simulink model "CEGR_TestBench_10kW_SimplifiedEGR_v01"  (R2025b)
settings: Solver=ode4  StartTime=0.0  StopTime=120  FixedStep=0.02  RelTol=1e-3
undefined symbols (not defined in the file): CaseBoundaryParam_simplified, CoolingCurveParam_simplified, dt_s_simplified, EGRInitialNode_simplified, PhysicalParam_simplified, StackInitialState_simplified, StackModelParam_simplified
settings Model: Creator=ADMIN  LastModifiedBy=ADMIN

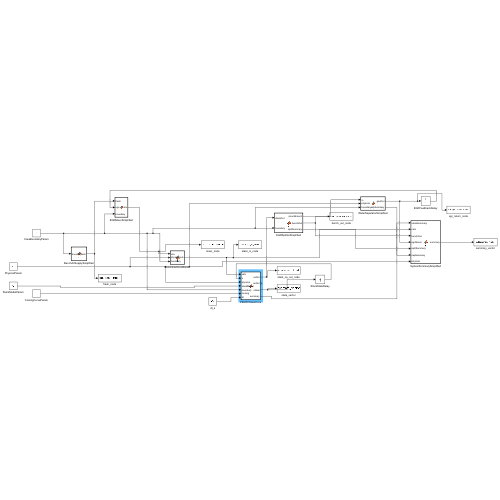
[thumbnail: Simulink's stored preview of the top-level diagram]
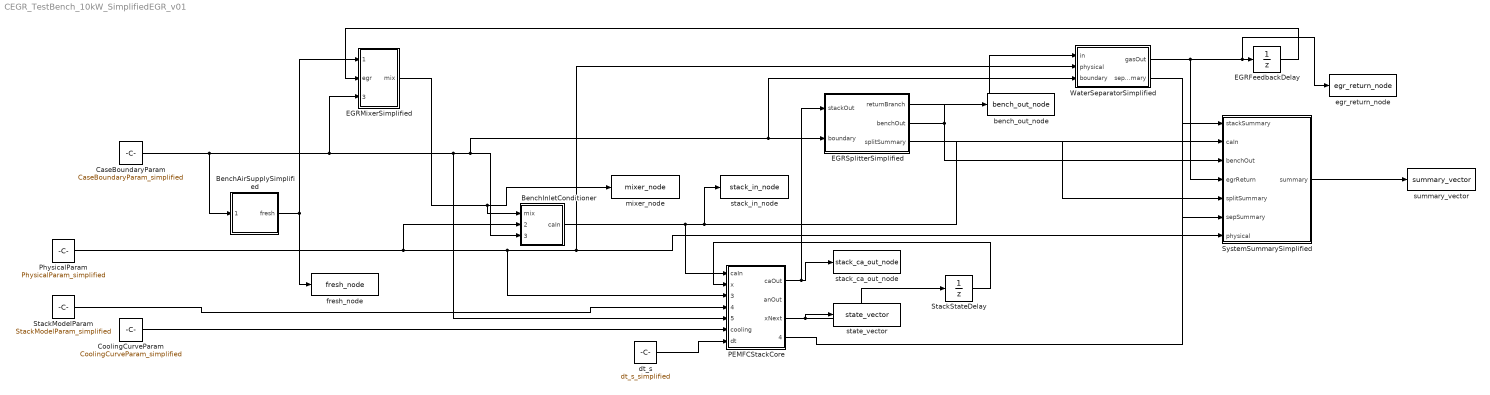
== system CEGR_TestBench_10kW_SimplifiedEGR_v01 ==
  BenchAirSupplySimplified : MATLAB Function  TreatAsAtomicUnit=on
  BenchInletConditioner : MATLAB Function  TreatAsAtomicUnit=on
  CaseBoundaryParam : Constant  Value=CaseBoundaryParam_simplified
  CoolingCurveParam : Constant  Value=CoolingCurveParam_simplified
  EGRFeedbackDelay : UnitDelay  InitialCondition=EGRInitialNode_simplified  SampleTime=dt_s_simplified
  EGRMixerSimplified : MATLAB Function  TreatAsAtomicUnit=on
  EGRSplitterSimplified : MATLAB Function  TreatAsAtomicUnit=on
  PEMFCStackCore : MATLAB Function  TreatAsAtomicUnit=on
  PhysicalParam : Constant  Value=PhysicalParam_simplified
  StackModelParam : Constant  Value=StackModelParam_simplified
  StackStateDelay : UnitDelay  InitialCondition=StackInitialState_simplified  SampleTime=dt_s_simplified
  SystemSummarySimplified : MATLAB Function  TreatAsAtomicUnit=on
  WaterSeparatorSimplified : MATLAB Function  TreatAsAtomicUnit=on
  bench_out_node : ToWorkspace  VariableName=bench_out_node  SaveFormat=Structure With Time
  dt_s : Constant  Value=dt_s_simplified
  egr_return_node : ToWorkspace  VariableName=egr_return_node  SaveFormat=Structure With Time
  fresh_node : ToWorkspace  VariableName=fresh_node  SaveFormat=Structure With Time
  mixer_node : ToWorkspace  VariableName=mixer_node  SaveFormat=Structure With Time
  stack_ca_out_node : ToWorkspace  VariableName=stack_ca_out_node  SaveFormat=Structure With Time
  stack_in_node : ToWorkspace  VariableName=stack_in_node  SaveFormat=Structure With Time
  state_vector : ToWorkspace  VariableName=state_vector  SaveFormat=Structure With Time
  summary_vector : ToWorkspace  VariableName=summary_vector  SaveFormat=Structure With Time
  wires:
  PhysicalParam/1 -> WaterSeparatorSimplified/2(physical), SystemSummarySimplified/7(physical), PEMFCStackCore/3(physical), BenchInletConditioner/2(physical)
  CaseBoundaryParam/1 -> PEMFCStackCore/5(boundary), EGRSplitterSimplified/2(boundary), WaterSeparatorSimplified/3(boundary), BenchInletConditioner/3(boundary), EGRMixerSimplified/3(boundary), BenchAirSupplySimplified/1(boundary)
  StackModelParam/1 -> PEMFCStackCore/4(stackModel)
  CoolingCurveParam/1 -> PEMFCStackCore/6(cooling)
  StackStateDelay/1 -> PEMFCStackCore/2(x)
  BenchAirSupplySimplified/1(fresh) -> EGRMixerSimplified/1(fresh), fresh_node/1
  EGRFeedbackDelay/1 -> EGRMixerSimplified/2(egr)
  EGRMixerSimplified/1(mix) -> mixer_node/1, BenchInletConditioner/1(mix)
  BenchInletConditioner/1(caIn) -> SystemSummarySimplified/2(caIn), stack_in_node/1, PEMFCStackCore/1(caIn)
  PEMFCStackCore/1(caOut) -> EGRSplitterSimplified/1(stackOut), stack_ca_out_node/1
  WaterSeparatorSimplified/1(gasOut) -> EGRFeedbackDelay/1, egr_return_node/1, SystemSummarySimplified/4(egrReturn)
  PEMFCStackCore/3(xNext) -> StackStateDelay/1, state_vector/1
  PEMFCStackCore/4(summary) -> SystemSummarySimplified/1(stackSummary)
  EGRSplitterSimplified/2(benchOut) -> bench_out_node/1, SystemSummarySimplified/3(benchOut)
  EGRSplitterSimplified/3(splitSummary) -> SystemSummarySimplified/5(splitSummary)
  WaterSeparatorSimplified/2(sepSummary) -> SystemSummarySimplified/6(sepSummary)
  SystemSummarySimplified/1(summary) -> summary_vector/1
  EGRSplitterSimplified/1(returnBranch) -> WaterSeparatorSimplified/1(in)
  dt_s/1 -> PEMFCStackCore/7(dt)

== matlab function CEGR_TestBench_10kW_SimplifiedEGR_v01/EGRMixerSimplified ==
  data: fresh input; mix output; egr input; boundary input
function mix = f(fresh, egr, boundary)
% EGRMixerSimplified
% 功能：把台架新鲜供气与延迟回流 EGR 混合，并生成目标入堆质量流量。
% 位置：BenchAirSupplySimplified 与 BenchInletConditioner 之间。
% 输入 fresh：新鲜供气 7x1 向量，fresh(1:4) 在此处按组分质量分数使用。
% 输入 egr：来自 EGRFeedbackDelay 的回流 7x1 向量，egr(1:4) 为可回流质量流量。
% 输入 boundary：CaseBoundaryParam_simplified，本模块使用 boundary(4) 入堆目标总质量流量。
% 输出 mix：7x1 混合气向量，mix(1:4) 为质量流量，供 BenchInletConditioner 使用。
%#codegen

mTarget = boundary(4);
assert(mTarget > 0);
assert(all(fresh(1:4) >= 0));
assert(all(egr(1:4) >= 0));
assert(fresh(5) >= -40 && fresh(5) <= 120 && fresh(6) > 0);

% 新鲜气输入来自 BenchAirSupplySimplified，前四项应能归一化为组分比例。
freshMassBasis = sum(fresh(1:4));
assert(freshMassBasis > 0);
freshFrac = fresh(1:4) / freshMassBasis;

% EGR 可用量取回流气相质量流量。液态水只作为组分携带，不用于决定回流气体替代量。
availableEgrGas = sum(egr(1:3));
egrTotalBasis = sum(egr(1:4));

% 最多让 EGR 替代 95% 的目标入堆流量，保留至少 5% 新鲜气补充。
% 这是当前简化模型的物理/数值边界，不是输入数据纠错。
egrToMix = min(availableEgrGas, 0.95 * mTarget);
freshMakeup = mTarget - egrToMix;

if egrToMix > 0
    assert(egrTotalBasis > 0);
    assert(egr(5) >= -40 && egr(5) <= 120 && egr(6) > 0);
    egrFrac = egr(1:4) / egrTotalBasis;
else
    egrFrac = zeros(4, 1);
end

mix = zeros(7, 1);
mix(1:4) = freshMakeup * freshFrac + egrToMix * egrFrac;
mixedMass = freshMakeup + egrToMix;
assert(mixedMass > 0);
mix(5) = (fresh(5) * freshMakeup + egr(5) * egrToMix) / mixedMass;
mix(6) = fresh(6);
mix(7) = double(mix(4) > 1e-12);
end

== matlab function CEGR_TestBench_10kW_SimplifiedEGR_v01/BenchAirSupplySimplified ==
  data: fresh output; boundary input
function fresh = f(boundary)
% BenchAirSupplySimplified
% 功能：把台架新鲜空气边界转换为模型统一气体向量 fresh。
% 位置：气路最外侧的新鲜供气端，输出进入 EGRMixerSimplified。
% 输入 boundary：CaseBoundaryParam_simplified 单工况边界向量。
%   boundary(2) = stack_in_p_abs_kPa，阴极入口绝压边界。
%   boundary(3) = stack_in_T_C，阴极入口温度边界。
%   boundary(5:7) = cathode_supply_wO2/wN2/wH2O，由台架供气 p/T/RH 换算得到的湿空气质量分数。
% 输出 fresh：7x1 气体向量，约定为 [O2; N2; H2O_vapor; H2O_liquid; T_C; p_kPa; wetFlag]。
% 注意：fresh(1:3) 在这里是归一化质量分数，不是质量流量；实际入堆总流量由后续混合器使用 boundary(4) 施加。
%#codegen

% 供气质量分数是输入边界，不能在模型里静默截断；负值应暴露为数据或映射错误。
wO2 = boundary(5);
wN2 = boundary(6);
wV = boundary(7);
assert(wO2 >= 0 && wN2 >= 0 && wV >= 0);

% 允许微小数值误差下的归一化，但质量分数和必须为正。
massFractionSum = wO2 + wN2 + wV;
assert(massFractionSum > 0);

% 新鲜供气支路不携带液态水，wetFlag=0 表示未发生冷凝/液水携带。
fresh = [
    wO2 / massFractionSum
    wN2 / massFractionSum
    wV / massFractionSum
    0
    boundary(3)
    boundary(2)
    0
    ];
end

== matlab function CEGR_TestBench_10kW_SimplifiedEGR_v01/BenchInletConditioner ==
  data: mix input; caIn output; physical input; boundary input
function caIn = f(mix, physical, boundary)
% BenchInletConditioner
% 功能：把混合器输出整理为电堆阴极入口气体向量 caIn。
% 位置：EGRMixerSimplified 与 PEMFCStackCore 之间，代表台架测得的入堆边界。
% 输入 mix：7x1 混合气向量，[O2; N2; H2O_vapor; H2O_liquid; T_C; p_kPa; wetFlag]。
% 输入 physical：通用物性向量，本模块使用 O2/N2/H2O 摩尔质量 physical(3:5)。
% 输入 boundary：CaseBoundaryParam_simplified，本模块使用 boundary(2) 入口绝压和 boundary(3) 入口温度。
% 输出 caIn：7x1 阴极入口向量，质量流量来自 mix，温度/压力强制采用实测入堆边界。
%#codegen

M_O2 = physical(3);
M_N2 = physical(4);
M_H2O = physical(5);
p = boundary(2);
T = boundary(3);

% 这些是硬输入/物性检查。异常值应暴露为参数或上游模块错误，不能静默修正。
assert(M_O2 > 0 && M_N2 > 0 && M_H2O > 0);
assert(p > 0);
assert(T >= -40 && T <= 120);
assert(all(mix(1:4) >= 0));

% 入口流量和组分沿用混合器输出；入口温压采用实验入堆边界。
caIn = mix;
caIn(5) = T;
caIn(6) = p;

% 依据入口温压计算可携带的饱和水蒸气质量流量。
% min(...,0.98*p) 是物理上限：水蒸气分压不能接近或超过总压。
pSat = min(sat_kPa(T), 0.98 * p);
nDry = caIn(1) / M_O2 + caIn(2) / M_N2;
assert(nDry > 0);
mVaporSat = pSat * nDry / (p - pSat) * M_H2O;

% 如果混合气在入口温压下超饱和，超出的水蒸气转为液态水。
if caIn(3) > mVaporSat
    caIn(4) = caIn(4) + caIn(3) - mVaporSat;
    caIn(3) = mVaporSat;
end
caIn(7) = double(caIn(4) > 1e-12);
end

function p = sat_kPa(T)
% Buck 饱和水蒸气压公式，T 单位 degC；调用前已检查适用温度范围。
p = 0.61121 * exp((18.678 - T / 234.5) * (T / (257.14 + T)));
end

== matlab function CEGR_TestBench_10kW_SimplifiedEGR_v01/PEMFCStackCore ==
  data: caIn input; caOut output; x input; physical input; stackModel input; anOut output; xNext output; summary output; boundary input; cooling input; dt input
function [caOut, anOut, xNext, summary] = f(caIn, x, physical, stackModel, boundary, cooling, dt)
% PEMFCStackCore
% 功能：电堆核心低维动态模型，计算阴极/阳极气体库存、膜水迁移、热平衡和单片电压。
% 输入 caIn：BenchInletConditioner 输出的阴极入口 7x1 向量，caIn(1:4) 为质量流量。
% 输入 x：StackStateDelay 反馈的状态向量 [mO2;mN2;mH2O_ca;mH2;mH2O_an;T_stack_C;mMem]。
% 输入 physical：物理常数向量 [R;F;M_O2;M_N2;M_H2O;M_H2;p_amb;T_amb]。
% 输入 stackModel：电堆结构、出口导纳、热参数、电压参数和膜水松弛参数。
% 输入 boundary：单工况边界；本模块使用电流、出口背压、阳极入口和冷却边界。
% 输入 cooling：冷却流量-换热系数曲线；dt：离散仿真步长。
% 输出 caOut/anOut：电堆阴极/阳极出口气体向量；输出 xNext：下一步状态；summary：诊断量。
%#codegen

% 参数解包。
R = physical(1); F = physical(2); M_O2 = physical(3); M_N2 = physical(4); M_H2O = physical(5); M_H2 = physical(6); pamb = physical(7); Tamb = physical(8);
N = stackModel(1); A = stackModel(2); Vca = stackModel(3); Van = stackModel(4); Kca = stackModel(5); Kan = stackModel(6); Cfc = stackModel(7); hCool = stackModel(8); hAmb = stackModel(9);
Eref = stackModel(10); Etemp = stackModel(11); theta1 = stackModel(12); theta2 = stackModel(13); theta3 = stackModel(14); theta4 = stackModel(15); sigmaPemCorrection = stackModel(16); Vtn = stackModel(17); tauMem = stackModel(18);
% 书籍活化极化经验式使用 theta1~theta4；欧姆项使用膜电导率公式。
% I_leak 固定为 0.01 A/cm2，只用于 log(j + I_leak) 避免零电流奇异。
jLeak = 0.01;
deltaCm = 0.0025; rhoMem = 1980.0; EW = 1.10;
I = boundary(1); pcBack = boundary(8); anFlow = boundary(12); anWH2 = boundary(13); anWV = boundary(14); panBack = boundary(15); Tcool = boundary(16); coolantFlow = boundary(17);

% 输入硬校验：这些是参数或边界错误，不能在核心模型里静默夹取。
assert(R > 0 && F > 0 && M_O2 > 0 && M_N2 > 0 && M_H2O > 0 && M_H2 > 0);
assert(pamb > 0 && Tamb >= -40 && Tamb <= 120);
assert(N > 0 && A > 0 && Vca > 0 && Van > 0 && Cfc > 0 && tauMem > 0);
assert(Kca >= 0 && Kan >= 0 && hCool >= 0 && hAmb >= 0);
assert(theta3 < 0 && theta4 >= 0 && jLeak >= 0);
assert(deltaCm > 0 && sigmaPemCorrection > 0 && rhoMem > 0 && EW > 0);
assert(I >= 0 && pcBack > 0 && panBack > 0 && anFlow > 0 && Tcool >= -40 && Tcool <= 120 && coolantFlow >= 0 && dt > 0);
assert(anWH2 >= 0 && anWH2 <= 1 && anWV >= 0 && anWV <= 1 && anWH2 + anWV <= 1.000001);
assert(numel(x) >= 6 && all(x(1:5) >= 0) && x(6) >= -40 && x(6) <= 120);
assert(all(caIn(1:4) >= 0) && caIn(5) >= -40 && caIn(5) <= 120 && caIn(6) > 0);
assert(sum(caIn(1:3)) > 0);

% 冷却换热系数：只有曲线启用且有效断点不少于 2 个时，才用流量插值覆盖默认 hCool。
hCoolEff = hCool;
nCool = floor((numel(cooling) - 1) / 2);
if nCool >= 2 && cooling(1) > 0.5
    hCoolEff = interp_hcool_flow(coolantFlow, cooling(2:1+nCool), cooling(2+nCool:1+2*nCool), hCool);
end

% 状态读取：正气体库存使用小正数下限只为避免除零；负状态已由上方断言拦截。
mO2 = max(x(1), 1e-12); mN2 = max(x(2), 1e-12); mV = x(3); mH2 = max(x(4), 1e-12); mVAn = x(5); T = x(6); TK = T + 273.15;
mMemPrev = 0;
if numel(x) >= 7
    mMemPrev = x(7);
end

% 阴极入口与反应源项。
mInCmd = sum(caIn(1:3)); mIn = mInCmd; wIn = caIn(1:3) / mInCmd;
mO2In = mIn * wIn(1); mN2In = mIn * wIn(2); mVIn = mIn * wIn(3);
mO2React = I * N / (4 * F) * M_O2; mH2React = I * N / (2 * F) * M_H2; mWater = I * N / (2 * F) * M_H2O;
lambdaO2 = (mO2In / M_O2) / max(I * N / (4 * F), 1e-12);
mH2In = anFlow * anWH2; mVAnIn = anFlow * anWV;
nInTot = mO2In / M_O2 + mN2In / M_N2 + mVIn / M_H2O;
pVInCa = caIn(6) * (mVIn / M_H2O) / max(nInTot, 1e-12);

% Pre 基准库存：先施加入堆流量、反应消耗和产水，但暂不施加跨膜水通量。
mO2Base = max(mO2 + dt * (mO2In - mO2React), 1e-12);
mN2Base = max(mN2 + dt * mN2In, 1e-12);
mVBaseAct = max(mV + dt * mVIn, 0);
mVBaseGas = max(mV + dt * (mVIn + mWater), 0);
mH2Base = max(mH2 + dt * (mH2In - mH2React), 1e-12);
mVAnBase = max(mVAn + dt * mVAnIn, 0);

% 膜含水量和跨膜水通量：使用同一时间步的 pre 水库存，而不是旧状态库存。
% mMem 与两侧 pre 水库存相互耦合，这里用固定 3 次 Picard 迭代近似求解，避免引入 Simulink 代数环。
A_m2 = A * 1e-4; delta_m = deltaCm * 0.01;
mMemMaxPos = mVAnBase / dt;
mMemMaxNeg = -mVBaseAct / dt;
mMem = min(max(mMemPrev, mMemMaxNeg), mMemMaxPos);
ps = sat_kPa(T);
lambdaCa = 0; lambdaAn = 0; lam = 0;
JDrag = 0; JDiff = 0; JNetRaw = 0;
nDragMol = 0; nDiffMol = 0; mDrag = 0; mDiff = 0; mMemRaw = 0; mMemTarget = 0;
for memIter = 1:3
    mVForMem = max(mVBaseAct + dt * mMem, 0);
    mVAnForMem = max(mVAnBase - dt * mMem, 0);
    pVPreMemBulk = mVForMem / M_H2O * R * TK / Vca / 1000;
    pVPreMem = 0.02 * pVInCa + 0.98 * pVPreMemBulk;
    pVAnPreMem = mVAnForMem / M_H2O * R * TK / Van / 1000;
    aCa = min(pVPreMem / ps, 3);
    aAn = min(pVAnPreMem / ps, 3);
    lambdaCa = lambda_eq(aCa); lambdaAn = lambda_eq(aAn); lam = 0.5 * (lambdaCa + lambdaAn);
    nDrag = max(0.0029 * lam^2 + 0.05 * lam, 0); D = membrane_diff(lam, TK);
    cMemCa = rhoMem / EW * lambdaCa; cMemAn = rhoMem / EW * lambdaAn;
    JDrag = nDrag * I / (F * A_m2); JDiff = D / delta_m * (cMemCa - cMemAn); JNetRaw = JDrag - JDiff;
    nDragMol = JDrag * A_m2 * N; nDiffMol = JDiff * A_m2 * N;
    mDrag = JDrag * A_m2 * N * M_H2O; mDiff = JDiff * A_m2 * N * M_H2O; mMemRaw = JNetRaw * A_m2 * N * M_H2O;
    mMemTarget = min(max(mMemRaw, mMemMaxNeg), mMemMaxPos);
    alpha = min(dt / max(tauMem, dt), 1);
    mMemRelax = mMemPrev + alpha * (mMemTarget - mMemPrev);
    mMem = min(max(mMemRelax, mMemMaxNeg), mMemMaxPos);
end
JNet = mMem / (A_m2 * N * M_H2O); mMemLimit = mMem - mMemRaw;

% 预出口库存：反应、入堆和跨膜水通量统一作用后的同一时间步 pre 状态。
mO2Pre = mO2Base; mN2Pre = mN2Base; mVPre = max(mVBaseGas + dt * mMem, 0);
mH2Pre = mH2Base; mVAnPre = max(mVAnBase - dt * mMem, 0);
% 出口前压力和等效出口流量：压差小于 0 时按无反向流处理；单步最多排出 95% 库存。
pO2Pre = mO2Pre / M_O2 * R * TK / Vca / 1000; pN2Pre = mN2Pre / M_N2 * R * TK / Vca / 1000; pVPre = mVPre / M_H2O * R * TK / Vca / 1000;
pCaPre = max(pO2Pre + pN2Pre + pVPre, pamb);
pH2Pre = mH2Pre / M_H2 * R * TK / Van / 1000; pVAnPre = mVAnPre / M_H2O * R * TK / Van / 1000; pAnPre = max(pH2Pre + pVAnPre, pamb);
gasCa = max(mO2Pre + mN2Pre + mVPre, 1e-12); wO2 = mO2Pre / gasCa; wN2 = mN2Pre / gasCa; wV = mVPre / gasCa;
mCaOutRaw = Kca * max(pCaPre - pcBack, 0) / (1 + Kca * max(pCaPre, 1e-6) * dt / gasCa);
mCaOut = min(mCaOutRaw, 0.95 * gasCa / dt);
gasAn = max(mH2Pre + mVAnPre, 1e-12); wH2 = mH2Pre / gasAn; wVAn = mVAnPre / gasAn;
mAnOutRaw = Kan * max(pAnPre - panBack, 0) / (1 + Kan * max(pAnPre, 1e-6) * dt / gasAn);
mAnOut = min(mAnOutRaw, 0.95 * gasAn / dt);

% 出口流量作用后的下一步库存。
mO2n = max(mO2Pre - dt * wO2 * mCaOut, 1e-12); mN2n = max(mN2Pre - dt * wN2 * mCaOut, 1e-12); mVnRaw = max(mVPre - dt * wV * mCaOut, 0);
mH2n = max(mH2Pre - dt * wH2 * mAnOut, 1e-12); mVAnnRaw = max(mVAnPre - dt * wVAn * mAnOut, 0);

% 电压模型：Nernst - 书籍经验活化损失 - 膜电导率欧姆损失。
% 当前实验电流范围内未呈现明显浓差极化拐点，因此 etaCon 暂置 0。
% 欧姆项中的 lambda 来自上方膜水计算得到的 lam，不从标定表另行输入。
j = max(I / A, 1e-9);
E = Eref - Etemp * (TK - 298.15) + R * TK / (2 * F) * log(max(pH2Pre * 1000, 1) / 101325 * sqrt(max(pO2Pre * 1000, 1) / 101325));
cO2Diag = max(1.97e-7 * max(pO2Pre * 1000, 1) * exp(498 / TK), 1e-12);
etaAct = theta1 + theta2 * TK + theta3 * TK * log(cO2Diag) + theta4 * TK * log(j + jLeak);
assert(etaAct >= 0);
sigmaPem0 = (0.005193 * lam - 0.00326) * exp(1268 * (1 / 303.15 - 1 / TK));
sigmaPem = sigmaPemCorrection * sigmaPem0;
assert(sigmaPem > 0);
RmArea = deltaCm / sigmaPem;
etaOhm = j * RmArea;
iLim = 0; etaCon = 0;
V = E - etaAct - etaOhm;

% 热平衡：T 表示入/出口平均电堆温度；方案 B 用 Tca_out = 2*T - Tca_in 估算阴极出口带热。
Pstack = I * V * N; Qgen = I * N * (Vtn - V); Qcool = hCoolEff * (T - Tcool); Qamb = hAmb * (T - Tamb); TcaOutHeat = 2 * T - caIn(5); Qgas = mCaOut * 1050 * (TcaOutHeat - caIn(5)) + mAnOut * 1050 * max(T - caIn(5), 0);
Qnet = Qgen - Qcool - Qamb - Qgas; Tn = T + dt * Qnet / Cfc;

% 饱和水蒸气库存裁剪：裁掉部分作为冷凝诊断量输出。
[mVn, liqDiag, psCaNext] = clip_vapor_inventory(mVnRaw, Vca, Tn, physical);
[mVAnn, liqAnDiag, psAnNext] = clip_vapor_inventory(mVAnnRaw, Van, Tn, physical);
phaseCa = (mVnRaw - mVn) / dt; phaseAn = (mVAnnRaw - mVAnn) / dt;

% 下一步分压、出口向量和诊断量：出口压力使用边界背压，不输出内部库存压力。
TKn = Tn + 273.15;
pO2Diag = mO2n / M_O2 * R * TKn / Vca / 1000; pN2Diag = mN2n / M_N2 * R * TKn / Vca / 1000; pVDiag = mVn / M_H2O * R * TKn / Vca / 1000; pCaDiag = max(pO2Diag + pN2Diag + pVDiag, pamb);
pH2Diag = mH2n / M_H2 * R * TKn / Van / 1000; pVAnDiag = mVAnn / M_H2O * R * TKn / Van / 1000; pAnDiag = max(pH2Diag + pVAnDiag, pamb);
xNext = [mO2n; mN2n; mVn; mH2n; mVAnn; Tn; mMem];
TcaOut = 2 * Tn - caIn(5); caOut = [wO2 * mCaOut; wN2 * mCaOut; wV * mCaOut; 0; TcaOut; pcBack; 0];
anOut = [wH2 * mAnOut; 0; wVAn * mAnOut; 0; Tn; panBack; 0];
nTot = max(mO2n / M_O2 + mN2n / M_N2 + mVn / M_H2O, 1e-12); xO2 = (mO2n / M_O2) / nTot; RH = pVDiag / max(sat_kPa(Tn), 1e-6);
nInTot = caIn(1) / M_O2 + caIn(2) / M_N2 + caIn(3) / M_H2O; xO2In = (caIn(1) / M_O2) / nInTot; pO2In = caIn(6) * xO2In; RHIn = (caIn(6) * (caIn(3) / M_H2O) / nInTot) / max(sat_kPa(caIn(5)), 1e-6);
resO2 = (mO2n - mO2) / dt - (mO2In - wO2 * mCaOut - mO2React); resN2 = (mN2n - mN2) / dt - (mN2In - wN2 * mCaOut);
resH2Ov = (mVn - mV) / dt - (mVIn - wV * mCaOut + mWater + mMem - phaseCa); resH2 = (mH2n - mH2) / dt - (mH2In - wH2 * mAnOut - mH2React); resH2OvAn = (mVAnn - mVAn) / dt - (mVAnIn - wVAn * mAnOut - mMem - phaseAn);
maxGasRes = max(abs([resO2, resN2, resH2Ov, resH2, resH2OvAn]));
summary = [I; V; Pstack; pO2Diag; pCaDiag; pH2Diag; pAnDiag; lam; Tn; xO2; RH; mMem; mO2React; mH2React; mWater; mCaOut; mAnOut; Cfc * (Tn - T) / dt - Qnet; pO2In; xO2In; RHIn; Qnet; resO2; resN2; resH2Ov; phaseCa; resH2; resH2OvAn; phaseAn; phaseCa + phaseAn; maxGasRes; Qgen; Qcool; Qamb; Qgas; E; etaAct; etaOhm; etaCon; lambdaO2; mIn; iLim; cO2Diag; mVIn; wV * mCaOut; mVAnIn; wVAn * mAnOut; liqDiag + liqAnDiag; lambdaCa; lambdaAn; nDragMol; nDiffMol; psCaNext; psAnNext; mVnRaw; mVAnnRaw; liqDiag; liqAnDiag; JDrag; JDiff; JNet; mDrag; mDiff; mMemRaw; mMemLimit; mMemTarget; tauMem];
end

function [mv, condensed, ps] = clip_vapor_inventory(mv0, V, T, physical)
% 将水蒸气库存限制在当前温度、体积下的饱和水蒸气库存以内。
R = physical(1); M_H2O = physical(5); TK = T + 273.15;
assert(V > 0 && TK > 0 && T >= -40 && T <= 120);
ps = sat_kPa(T); mSat = ps * 1000 * V * M_H2O / (R * TK);
if mv0 > mSat
    mv = mSat; condensed = mv0 - mSat;
else
    mv = mv0; condensed = 0;
end
end

function p = sat_kPa(T)
% Buck 饱和水蒸气压公式，T 单位 degC；调用前不再静默夹取温度。
assert(T >= -40 && T <= 120);
p = 0.61121 * exp((18.678 - T / 234.5) * (T / (257.14 + T)));
end

function lambda = lambda_eq(a)
% Springer 型膜含水量经验关系。a>1 时按线性外推处理。
assert(a >= 0);
if a <= 1
    lambda = 0.043 + 17.81 * a - 39.85 * a^2 + 36 * a^3;
else
    lambda = 14 + 1.4 * (a - 1);
end
end

function D = membrane_diff(lambda, TK)
% 膜水扩散系数经验式。lambda 分段来自常见 PEM 膜水扩散近似。
assert(lambda >= 0 && TK > 0);
if lambda < 2
    d0 = 1e-10;
elseif lambda < 3
    d0 = 1e-10 * (1 + 2 * (lambda - 2));
elseif lambda < 4.5
    d0 = 1e-10 * (3 - 1.167 * (lambda - 3));
else
    d0 = 1.25e-10;
end
D = d0 * exp(2416 * (1 / 303 - 1 / TK));
end

function h = interp_hcool_flow(flow, bp, hv, hFallback)
% 冷却流量断点插值；无效断点被忽略，超出断点范围时取端点值。
n = 0;
for k = 1:numel(bp)
    if bp(k) > 0 && hv(k) > 0
        n = n + 1;
    end
end
if n < 2
    h = hFallback; return;
end
b = zeros(n, 1); v = zeros(n, 1); j = 0;
for k = 1:numel(bp)
    if bp(k) > 0 && hv(k) > 0
        j = j + 1; b(j) = bp(k); v(j) = hv(k);
    end
end
if flow <= b(1)
    h = v(1); return;
end
if flow >= b(n)
    h = v(n); return;
end
h = v(n);
for k = 1:n-1
    if flow >= b(k) && flow <= b(k+1)
        a = (flow - b(k)) / max(b(k+1) - b(k), 1e-9);
        h = v(k) + a * (v(k+1) - v(k)); return;
    end
end
end

== matlab function CEGR_TestBench_10kW_SimplifiedEGR_v01/EGRSplitterSimplified ==
  data: stackOut input; returnBranch output; boundary input; benchOut output; splitSummary output
function [returnBranch, benchOut, splitSummary] = f(stackOut, boundary)
% EGRSplitterSimplified
% 功能：按工况 EGR 分流比例，把电堆阴极出口气体分成回流支路和台架外排支路。
% 输入 stackOut：来自 PEMFCStackCore.caOut 的 7x1 阴极出口向量，stackOut(1:4) 为质量流量。
% 输入 boundary：CaseBoundaryParam_simplified，本模块使用 boundary(11) 作为 EGR 分流比例。
% 输出 returnBranch：进入 WaterSeparatorSimplified 的回流支路；benchOut：台架外排支路。
% 输出 splitSummary：[r; m_return_gas; m_bench_out_gas; m_stack_out_gas; m_stack_liq; m_return_liq; m_bench_liq]。
%#codegen

r = boundary(11);
assert(r >= 0 && r <= 0.95);
assert(all(stackOut(1:4) >= 0));
assert(stackOut(5) >= -40 && stackOut(5) <= 120 && stackOut(6) > 0);

% 回流支路和外排支路继承电堆出口温度、压力和组分格式，只按质量流量分配。
returnBranch = stackOut;
returnBranch(1:4) = r * stackOut(1:4);
returnBranch(7) = double(returnBranch(4) > 1e-12);

benchOut = stackOut;
benchOut(1:4) = (1 - r) * stackOut(1:4);
benchOut(7) = double(benchOut(4) > 1e-12);

% 守恒诊断：气相只统计 O2/N2/H2O_vapor，液态水单独列出。
mStackOutGas = sum(stackOut(1:3));
mReturnGas = sum(returnBranch(1:3));
mBenchOutGas = sum(benchOut(1:3));
splitSummary = [
    r
    mReturnGas
    mBenchOutGas
    mStackOutGas
    stackOut(4)
    returnBranch(4)
    benchOut(4)
    ];
end

== matlab function CEGR_TestBench_10kW_SimplifiedEGR_v01/WaterSeparatorSimplified ==
  data: in input; gasOut output; physical input; sepSummary output; boundary input
function [gasOut, sepSummary] = f(in, physical, boundary)
%#codegen
% WaterSeparatorSimplified：EGR 回流支路水分离器。
% 输入 in 来自 EGRSplitterSimplified.returnBranch，in(1:3) 为 O2/N2/H2O 气相质量流量，in(4) 为液态水流量，in(5:6) 为上游温度和压力。
% 本模块使用 separator_T_C=boundary(9) 和 separator_p_abs_kPa=boundary(10) 覆盖分离器出口气相温压。
% 计算内容为：按分离器温压下的饱和水汽容量冷凝超额水汽，并把入口液态水和冷凝水汇入 drain。
% 输出 gasOut 为分离后的气相回流，进入 EGRFeedbackDelay 后再进入 EGRMixerSimplified；sepSummary 记录排水、冷凝和出口气相状态。

M_O2 = physical(3);
M_N2 = physical(4);
M_H2O = physical(5);

assert(M_O2 > 0 && M_N2 > 0 && M_H2O > 0);
assert(all(in(1:4) >= 0));
assert(in(6) > 0);
assert(in(5) >= -40 && in(5) <= 120);

T = boundary(9);
p = boundary(10);
assert(T >= -40 && T <= 120);
assert(p > 0);

gasOut = in;
gasOut(5) = T;
gasOut(6) = p;
gasOut(7) = 0;

dryMolarFlow = gasOut(1) / M_O2 + gasOut(2) / M_N2;
vaporMolarFlow = gasOut(3) / M_H2O;
gasMolarFlow = dryMolarFlow + vaporMolarFlow;

if gasMolarFlow <= 0
    % 无 EGR 气相回流时，不人为制造微小干气；可能存在的入口液态水直接排出。
    condensed = 0;
    drain = gasOut(4);
    gasOut(1:4) = 0;
    rhOut = 0;
else
    % 有气相回流时必须含有干气，否则无法用湿空气饱和关系定义水汽容量。
    assert(dryMolarFlow > 0);
    ps = min(sat_kPa(T), 0.98 * p);
    mSat = ps * dryMolarFlow / (p - ps) * M_H2O;

    % 冷凝量不能为负；未超过饱和容量时不发生冷凝。
    condensed = max(gasOut(3) - mSat, 0);
    gasOut(3) = gasOut(3) - condensed;
    drain = gasOut(4) + condensed;
    gasOut(4) = 0;
    rhOut = rel_hum(gasOut, M_O2, M_N2, M_H2O);
end

sepSummary = [drain; condensed; in(4); rhOut; T; p; sum(gasOut(1:3))];
end

function rh = rel_hum(node, M_O2, M_N2, M_H2O)
nV = node(3) / M_H2O;
nTot = node(1) / M_O2 + node(2) / M_N2 + nV;
assert(nV >= 0 && nTot > 0);
rh = node(6) * nV / nTot / sat_kPa(node(5));
end

function pSat = sat_kPa(T)
assert(T >= -40 && T <= 120);
pSat = 0.61121 * exp((18.678 - T / 234.5) * (T / (257.14 + T)));
end

== matlab function CEGR_TestBench_10kW_SimplifiedEGR_v01/SystemSummarySimplified ==
  data: stackSummary input; summary output; caIn input; benchOut input; egrReturn input; splitSummary input; sepSummary input; physical input
function summary = f(stackSummary, caIn, benchOut, egrReturn, splitSummary, sepSummary, physical)
%#codegen
% SystemSummarySimplified：系统级诊断向量汇总模块。
% 本模块不参与气体、水、热、电压计算，只把各模块诊断量按固定顺序拼接。
% summary(1:67)  = PEMFCStackCore.stackSummary。
% summary(68:71) = 系统级入口氧摩尔分数、入口气相流量、EGR 回流气相流量、台架外排气相流量。
% summary(72:78) = EGRSplitterSimplified.splitSummary。
% summary(79:85) = WaterSeparatorSimplified.sepSummary。
% 脚本中的 summary_vector 索引依赖这个顺序，修改前必须同步更新脚本和说明文档。

M_O2 = physical(3);
M_N2 = physical(4);
M_H2O = physical(5);

assert(numel(stackSummary) == 67);
assert(numel(caIn) == 7);
assert(numel(benchOut) == 7);
assert(numel(egrReturn) == 7);
assert(numel(splitSummary) == 7);
assert(numel(sepSummary) == 7);
assert(M_O2 > 0 && M_N2 > 0 && M_H2O > 0);
assert(all(caIn(1:3) >= 0));
assert(all(benchOut(1:3) >= 0));
assert(all(egrReturn(1:3) >= 0));

nO2In = caIn(1) / M_O2;
nIn = nO2In + caIn(2) / M_N2 + caIn(3) / M_H2O;
assert(nIn > 0);

xO2In = nO2In / nIn;
mIn = sum(caIn(1:3));
mEgr = sum(egrReturn(1:3));
mBenchOut = sum(benchOut(1:3));

summary = [stackSummary; xO2In; mIn; mEgr; mBenchOut; splitSummary; sepSummary];
end
